simulink model "RPBC560"  (Simulink 8.8)
settings: Solver=ode45  StartTime=0.0  StopTime=pi  RelTol=1e-3  EnableMultiTasking=on
values from neighbouring files (symbols this model uses):
  A1 = 1    [setupRPBC.m]
  A2 = 0.25    [setupRPBC.m]
  A3 = 0.5    [setupRPBC.m]
  A_Matrix = [A_Matrix a]    [systemident.m]
  b1 = 0    [setupRPBC.m]
  b2 = 0    [setupRPBC.m]
  b3 = -pi/2    (= -1.57079632679)    [setupRPBC.m]
  B_Matrix = [B_Matrix B_e]    [systemident.m]
  w1 = 2    [setupRPBC.m]
  w2 = 2    [setupRPBC.m]
  w3 = 2    [setupRPBC.m]
  Z0 = [0;0;0;0;-pi/2;0]    [setupRPBC.m]
undefined symbols (not defined in the file or in its folder): RPBCpuma, statederPUMA3
settings Model: Creator=rhanz  LastModifiedBy=R4hul  ExtModeAutoUpdateStatusClock=off
settings OptimizationCC: ExpressionDepthLimit=2147483647  InitFltsAndDblsToZero=on
settings DebuggingCC: SaveWithParameterizedLinksMsg=none  SignalResolutionControl=TryResolveAllWithWarning  MultiTaskDSMMsg=warning  MultiTaskCondExecSysMsg=none
settings GRTTargetCC: TargetFcnLib=ansi_tfl_tmw.mat

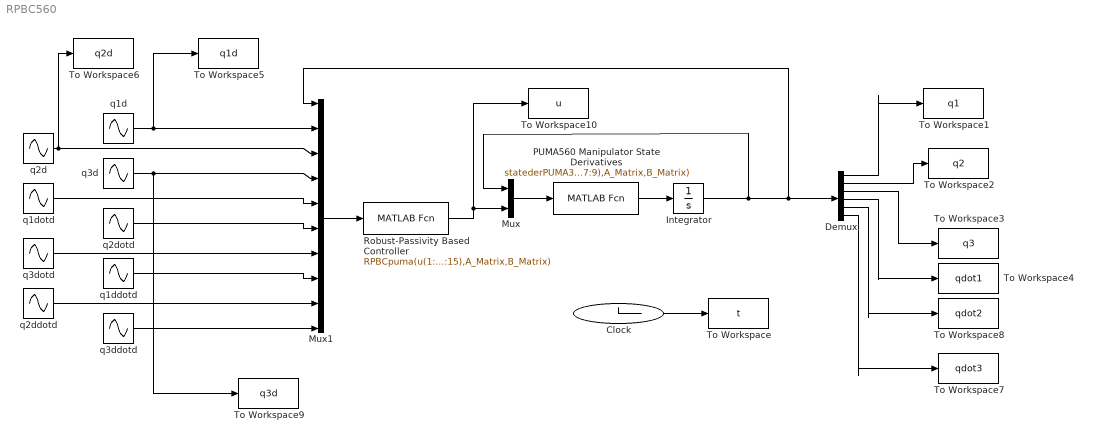
== system RPBC560 ==
  Clock : Clock
  Demux : Demux  Outputs=6
  Integrator : Integrator  InitialCondition=Z0
  Mux : Mux  Inputs=2
  Mux1 : Mux  Inputs=10
  PUMA560 Manipulator State Derivatives : MATLABFcn  MATLABFcn=statederPUMA3(u(1:6),u(7:9),A_Matrix,B_Matrix)  OutputDimensions=6
  Robust-Passivity Based Controller : MATLABFcn  MATLABFcn=RPBCpuma(u(1:6),u(7:15),A_Matrix,B_Matrix)  OutputDimensions=3
  To Workspace : ToWorkspace  VariableName=t  SampleTime=-1
  To Workspace1 : ToWorkspace  VariableName=q1  SampleTime=-1
  To Workspace10 : ToWorkspace  VariableName=u  SampleTime=-1
  To Workspace2 : ToWorkspace  VariableName=q2  SampleTime=-1
  To Workspace3 : ToWorkspace  VariableName=q3  SampleTime=-1
  To Workspace4 : ToWorkspace  VariableName=qdot1  SampleTime=-1
  To Workspace5 : ToWorkspace  VariableName=q1d  SampleTime=-1
  To Workspace6 : ToWorkspace  VariableName=q2d  SampleTime=-1
  To Workspace7 : ToWorkspace  VariableName=qdot3  SampleTime=-1
  To Workspace8 : ToWorkspace  VariableName=qdot2  SampleTime=-1
  To Workspace9 : ToWorkspace  VariableName=q3d  SampleTime=-1
  q1d : Sin  Amplitude=A1  Bias=b1  Frequency=w1  SampleTime=0
  q1ddotd : Sin  Amplitude=A1*w1^2  Frequency=w1  Phase=pi  SampleTime=0
  q1dotd : Sin  Amplitude=A1*w1  Frequency=w1  Phase=pi/2  SampleTime=0
  q2d : Sin  Amplitude=A2  Bias=b2  Frequency=w2  SampleTime=0
  q2ddotd : Sin  Amplitude=A2*w2^2  Frequency=w2  Phase=pi  SampleTime=0
  q2dotd : Sin  Amplitude=A2*w2  Frequency=w2  Phase=pi/2  SampleTime=0
  q3d : Sin  Amplitude=A3  Bias=b3  Frequency=w3  SampleTime=0
  q3ddotd : Sin  Amplitude=A3*w3^2  Frequency=w3  Phase=pi  SampleTime=0
  q3dotd : Sin  Amplitude=A3*w3  Frequency=w3  Phase=pi/2  SampleTime=0
  wires:
  PUMA560 Manipulator State Derivatives/1 -> Integrator/1
  Integrator/1 -> Mux/1, Demux/1, Mux1/1
  Mux/1 -> PUMA560 Manipulator State Derivatives/1
  Clock/1 -> To Workspace/1
  Demux/1 -> To Workspace1/1
  Demux/3 -> To Workspace3/1
  Demux/4 -> To Workspace4/1
  Mux1/1 -> Robust-Passivity Based Controller/1
  q1d/1 -> Mux1/2, To Workspace5/1
  q2d/1 -> Mux1/3, To Workspace6/1
  q3d/1 -> Mux1/4, To Workspace9/1
  q1dotd/1 -> Mux1/5
  q2dotd/1 -> Mux1/6
  q3dotd/1 -> Mux1/7
  q1ddotd/1 -> Mux1/8
  q2ddotd/1 -> Mux1/9
  q3ddotd/1 -> Mux1/10
  Demux/2 -> To Workspace2/1
  Demux/5 -> To Workspace8/1
  Demux/6 -> To Workspace7/1
  Robust-Passivity Based Controller/1 -> To Workspace10/1, Mux/2
